simulink model "TJA_Model"  (R2025a)
settings: Solver=FixedStepDiscrete  StartTime=0.0  StopTime=1.0  FixedStep=0.01  RelTol=1e-3
settings Model: DataDictionary=TJA_Data.sldd  Creator=nikul  LastModifiedBy=nikul
settings OptimizationCC: DefaultParameterBehavior=Inlined  EnhancedBackFolding=on  PassReuseOutputArgsAs=Individual arguments  ZeroExternalMemoryAtStartup=off  ZeroInternalMemoryAtStartup=off  OptimizeBlockOrder=speed  DifferentSizesBufferReuse=on  OptimizationCustomize=off  EfficientTunableParamExpr=on
settings DebuggingCC: ParameterTunabilityLossMsg=error
settings SFSimCC: MATLABDynamicMemAlloc=off
settings RTWCC: SystemTargetFile=ert.tlc  TemplateMakefile=ert_default_tmf  Description=Embedded Coder
settings CodeAppCC: ForceParamTrailComments=on  IgnoreCustomStorageClasses=off  OperatorAnnotations=on  SimulinkDataObjDesc=on  SFDataObjDesc=on  InsertBlockDesc=on
settings ERTTargetCC: ExtModeTransport=0.0  ExtModeStaticAlloc=off  ExtModeMexFile=ext_comm  ExtModeIntrfLevel=Level1  ERTCustomFileTemplate=example_file_process.tlc  TargetLangStandard=C99 (ISO)  GenerateSampleERTMain=on
settings ConfigComp: CovEnable=on  RecordCoverage=on  CovMetricSettings=dcmwe  CovModelRefEnable=on

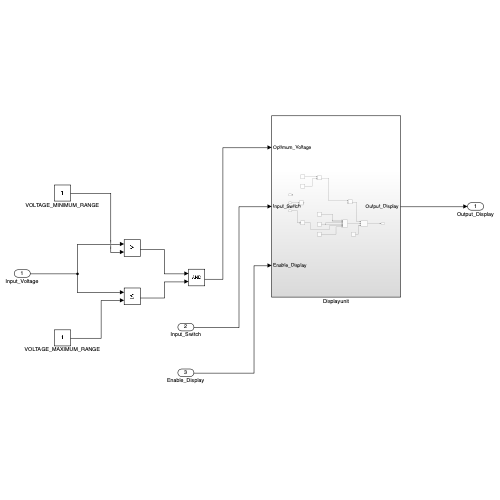
[thumbnail: Simulink's stored preview of the top-level diagram]
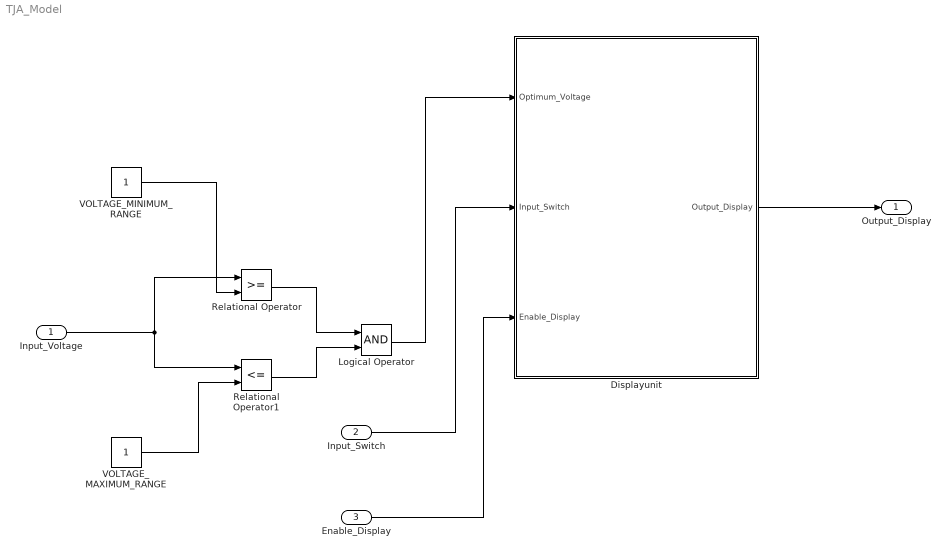
== system TJA_Model ==
  Input_Voltage : Inport
  Input_Switch : Inport  Port=2
  Enable_Display : Inport  Port=3
  Displayunit : Subsystem
  Logical Operator : Logic  AllPortsSameDT=off  OutDataTypeStr=boolean
  Relational Operator : RelationalOperator  OutDataTypeStr=boolean  RndMeth=Simplest  InputSameDT=off
  Relational Operator1 : RelationalOperator  Operator=<=  OutDataTypeStr=boolean  RndMeth=Simplest  InputSameDT=off
  VOLTAGE_MAXIMUM_RANGE : Constant
  VOLTAGE_MINIMUM_RANGE : Constant
  Output_Display : Outport
  wires:
  Input_Voltage/1 -> Relational Operator1/1, Relational Operator/1
  VOLTAGE_MINIMUM_RANGE/1 -> Relational Operator/2
  VOLTAGE_MAXIMUM_RANGE/1 -> Relational Operator1/2
  Relational Operator/1 -> Logical Operator/1
  Relational Operator1/1 -> Logical Operator/2
  Logical Operator/1 -> Displayunit/1(Optimum_Voltage)
  Input_Switch/1 -> Displayunit/2(Input_Switch)
  Enable_Display/1 -> Displayunit/3(Enable_Display)
  Displayunit/1(Output_Display) -> Output_Display/1

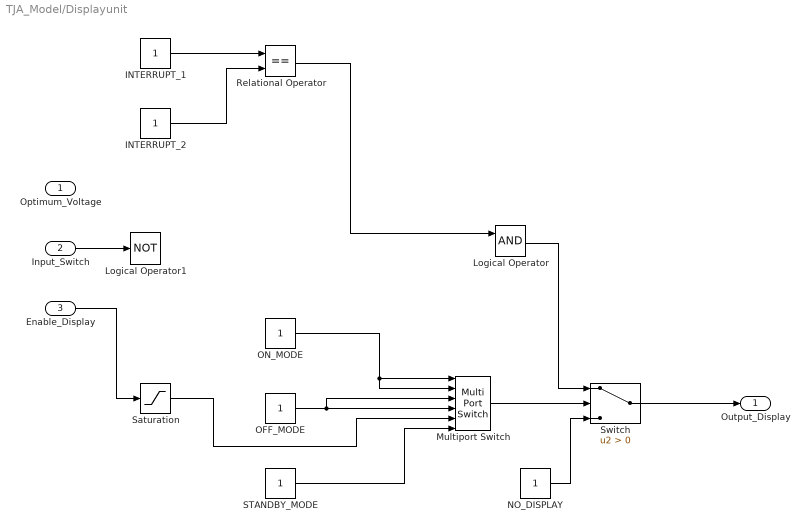
== system TJA_Model/Displayunit ==
  Optimum_Voltage : Inport
  Input_Switch : Inport  Port=2
  Enable_Display : Inport  Port=3
  INTERRUPT_1 : Constant
  INTERRUPT_2 : Constant
  Logical Operator : Logic  AllPortsSameDT=off  OutDataTypeStr=boolean
  Logical Operator1 : Logic  Operator=NOT  AllPortsSameDT=off  OutDataTypeStr=boolean
  Multiport Switch : MultiPortSwitch  Inputs=5  SaturateOnIntegerOverflow=off  InputSameDT=off
  NO_DISPLAY : Constant
  OFF_MODE : Constant
  ON_MODE : Constant
  Relational Operator : RelationalOperator  Operator===  OutDataTypeStr=boolean  RndMeth=Simplest  InputSameDT=off
  STANDBY_MODE : Constant
  Saturation : Saturate  UpperLimit=7  LowerLimit=0
  Switch : Switch  Criteria=u2 > Threshold  SaturateOnIntegerOverflow=off  InputSameDT=off
  Output_Display : Outport
  wires:
  Enable_Display/1 -> Saturation/1
  ON_MODE/1 -> Multiport Switch/2, Multiport Switch/1
  OFF_MODE/1 -> Multiport Switch/4, Multiport Switch/3
  STANDBY_MODE/1 -> Multiport Switch/6
  Saturation/1 -> Multiport Switch/5
  Input_Switch/1 -> Logical Operator1/1
  INTERRUPT_1/1 -> Relational Operator/1
  INTERRUPT_2/1 -> Relational Operator/2
  Relational Operator/1 -> Logical Operator/1
  Multiport Switch/1 -> Switch/2
  Logical Operator/1 -> Switch/1
  NO_DISPLAY/1 -> Switch/3
  Switch/1 -> Output_Display/1
